simulink model "ACD"  (R2022b)
settings: Solver=VariableStepAuto  StartTime=0.0  StopTime=10  FixedStep=0.002  MaxStep=0.2  RelTol=1e-3
libraries: simulink x1, simulink_extras x1
settings Model: Creator=beikuzi  LastModifiedBy=beikuzi

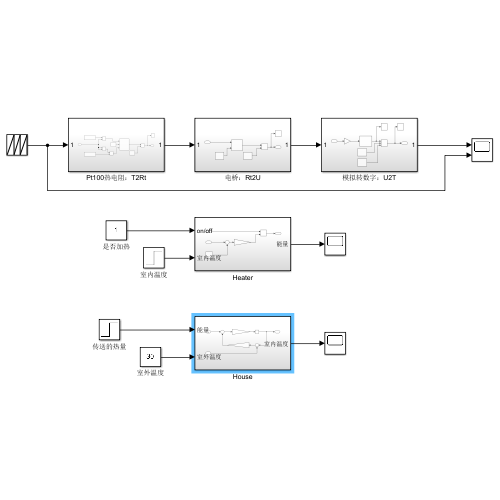
[thumbnail: Simulink's stored preview of the top-level diagram]
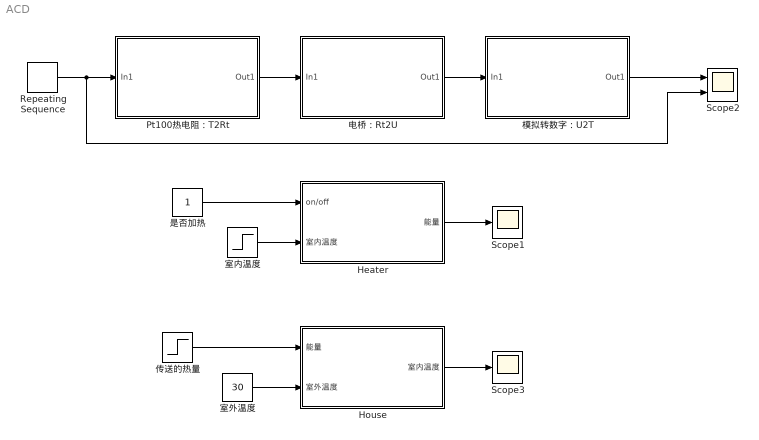
== system ACD ==
  Heater : Subsystem
  House : Subsystem
  Pt100热电阻：T2Rt : Subsystem
  Repeating Sequence : simulink/Sources/Repeating Sequence  rep_seq_t=[0 12]  rep_seq_y=[0 120]
  Scope1 : Scope
  Scope2 : Scope  NumInputPorts=2
  Scope3 : Scope
  传送的热量 : Step  Time=0  After=30  SampleTime=0
  室内温度 : Step  Time=0  After=30  SampleTime=0
  室外温度 : Constant  Value=30
  是否加热 : Constant
  模拟转数字：U2T : Subsystem
  电桥：Rt2U : Subsystem
  wires:
  Pt100热电阻：T2Rt/1(Out1) -> 电桥：Rt2U/1(In1)
  电桥：Rt2U/1(Out1) -> 模拟转数字：U2T/1(In1)
  模拟转数字：U2T/1(Out1) -> Scope2/1
  Heater/1(能量) -> Scope1/1
  是否加热/1 -> Heater/1(on/off)
  室内温度/1 -> Heater/2(室内温度)
  Repeating Sequence/1 -> Scope2/2, Pt100热电阻：T2Rt/1(In1)
  House/1(室内温度) -> Scope3/1
  室外温度/1 -> House/2(室外温度)
  传送的热量/1 -> House/1(能量)

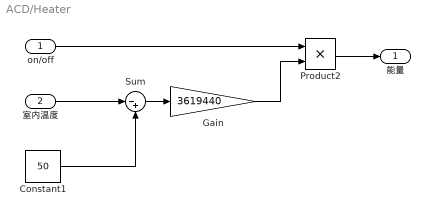
== system ACD/Heater ==
  on/off : Inport  OutMin=[0]  OutMax=[1]
  室内温度 : Inport  Port=2
  Constant1 : Constant  Value=50
  Gain : Gain  Gain=3619440
  Product2 : Product
  Sum : Sum  Inputs=|-+
  能量 : Outport
  wires:
  室内温度/1 -> Sum/1
  Constant1/1 -> Sum/2
  Sum/1 -> Gain/1
  on/off/1 -> Product2/1
  Gain/1 -> Product2/2
  Product2/1 -> 能量/1

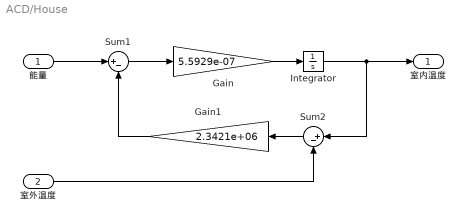
== system ACD/House ==
  能量 : Inport  OutMin=[0]  OutMax=[1]
  室外温度 : Inport  Port=2
  Gain : Gain  Gain=5.5929e-07
  Gain1 : Gain  Gain=2.3421e+06
  Integrator : Integrator  InitialCondition=20
  Sum1 : Sum  Inputs=|+-
  Sum2 : Sum  Inputs=|+-
  室内温度 : Outport
  wires:
  室外温度/1 -> Sum2/2
  能量/1 -> Sum1/1
  Sum1/1 -> Gain/1
  Sum2/1 -> Gain1/1
  Gain1/1 -> Sum1/2
  Gain/1 -> Integrator/1
  Integrator/1 -> Sum2/1, 室内温度/1

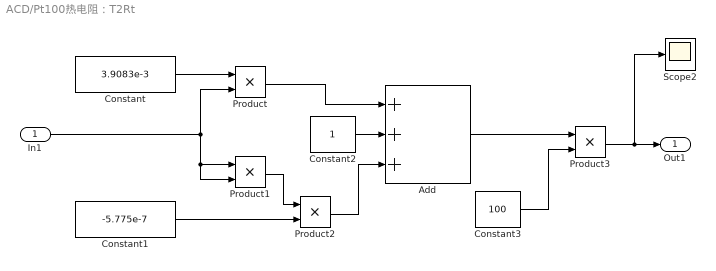
== system ACD/Pt100热电阻：T2Rt ==
  In1 : Inport
  Add : Sum  Inputs=+++
  Constant : Constant  Value=3.9083e-3
  Constant1 : Constant  Value=-5.775e-7
  Constant2 : Constant
  Constant3 : Constant  Value=100
  Product{,1..3} (4 alike) : Product
  Scope2 : Scope
  Out1 : Outport
  wires:
  In1/1 -> Product/2, Product1/2, Product1/1
  Constant/1 -> Product/1
  Constant1/1 -> Product2/2
  Product1/1 -> Product2/1
  Product/1 -> Add/1
  Product2/1 -> Add/3
  Constant2/1 -> Add/2
  Product3/1 -> Scope2/1, Out1/1
  Add/1 -> Product3/1
  Constant3/1 -> Product3/2

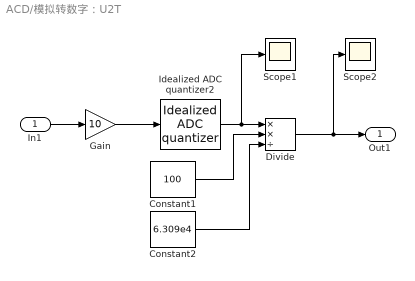
== system ACD/模拟转数字：U2T ==
  In1 : Inport
  Constant1 : Constant  Value=100
  Constant2 : Constant  Value=6.309e4
  Divide : Product  Inputs=**/
  Gain : Gain  Gain=10
  Idealized ADC quantizer2 : simulink_extras/Additional Discrete/Idealized ADC quantizer  NumberOfConverterBits=16  Vmin=0  Vmax=5  OutputDataType=int32  OutputNegativeValues=off
  Scope1 : Scope
  Scope2 : Scope
  Out1 : Outport
  wires:
  Idealized ADC quantizer2/1 -> Scope1/1, Divide/1
  Constant1/1 -> Divide/2
  Constant2/1 -> Divide/3
  Divide/1 -> Scope2/1, Out1/1
  In1/1 -> Gain/1
  Gain/1 -> Idealized ADC quantizer2/1

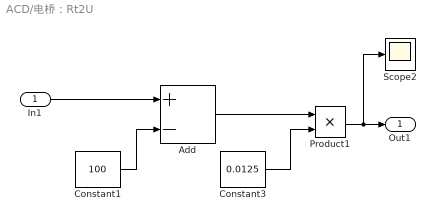
== system ACD/电桥：Rt2U ==
  In1 : Inport
  Add : Sum  Inputs=+-
  Constant1 : Constant  Value=100
  Constant3 : Constant  Value=0.0125
  Product1 : Product
  Scope2 : Scope
  Out1 : Outport
  wires:
  In1/1 -> Add/1
  Constant1/1 -> Add/2
  Add/1 -> Product1/1
  Constant3/1 -> Product1/2
  Product1/1 -> Scope2/1, Out1/1
